simulink model "p21"  (R2016b)
settings: Solver=VariableStepAuto  StartTime=0.0  StopTime=10.0  RelTol=1e-3
values from neighbouring files (symbols this model uses):
  b = 3.5077e-6    (= 3.5077e-06)    [p2_2_1.m]
  J = 3.2284e-5    (= 3.2284e-05)    [p2_2_1.m]
  K = 0.0274    [p2_2_1.m]
undefined symbols (not defined in the file or in its folder): L, R
settings Model: Creator=ASUS  LastModifiedBy=ASUS

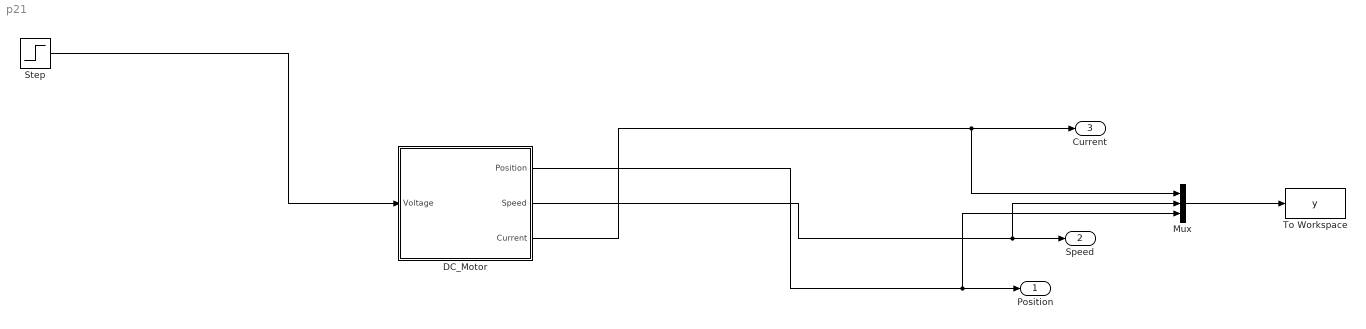
== system p21 ==
  DC_Motor : Subsystem
  Mux : Mux  Inputs=3
  Step : Step  SampleTime=0
  To Workspace : ToWorkspace  VariableName=y  SampleTime=-1
  Position : Outport
  Speed : Outport  Port=2
  Current : Outport  Port=3
  wires:
  Step/1 -> DC_Motor/1(Voltage)
  DC_Motor/1(Position) -> Mux/3, Position/1
  DC_Motor/2(Speed) -> Mux/2, Speed/1
  DC_Motor/3(Current) -> Mux/1, Current/1
  Mux/1 -> To Workspace/1

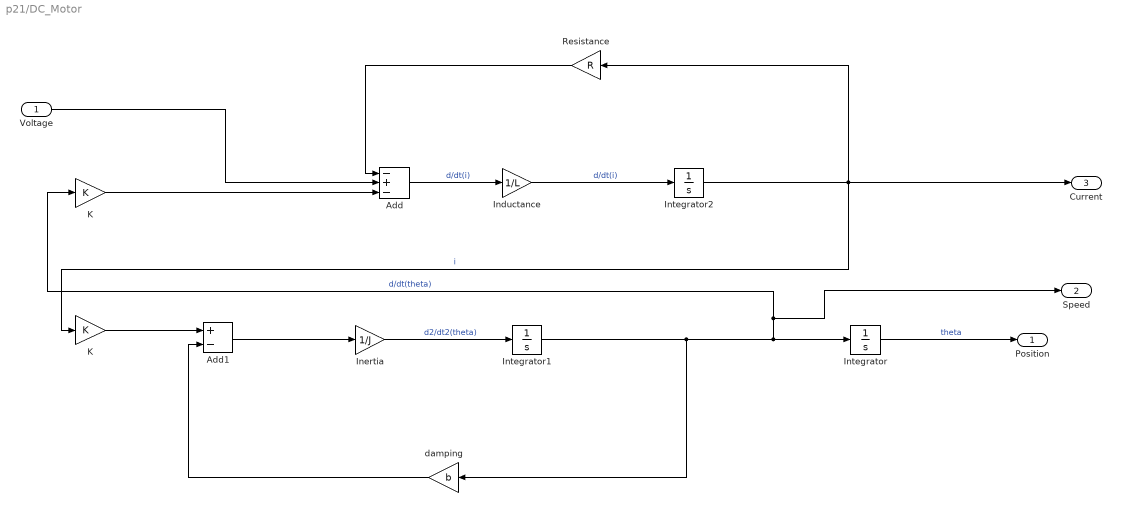
== system p21/DC_Motor ==
  Voltage : Inport
  Add : Sum  Inputs=-+-
  Add1 : Sum  Inputs=+-
  Inductance : Gain  Gain=1/L
  Inertia : Gain  Gain=1/J
  Integrator : Integrator
  Integrator1 : Integrator
  Integrator2 : Integrator
  K : Gain  Gain=K
  "K " : Gain  Gain=K
  Resistance : Gain  Gain=R
  damping : Gain  Gain=b
  Position : Outport
  Speed : Outport  Port=2
  Current : Outport  Port=3
  wires:
  Integrator2/1 -> Current/1, Resistance/1, "K "/1  "i"
  Integrator1/1 -> damping/1, Speed/1, K/1, Integrator/1  "d/dt(theta)"
  Inductance/1 -> Integrator2/1  "d/dt(i)"
  Inertia/1 -> Integrator1/1  "d2/dt2(theta)"
  Integrator/1 -> Position/1  "theta"
  K/1 -> Add/3
  damping/1 -> Add1/2
  Add1/1 -> Inertia/1
  Add/1 -> Inductance/1  "d/dt(i)"
  Resistance/1 -> Add/1
  "K "/1 -> Add1/1
  Voltage/1 -> Add/2
